simulink model "geometric_control_template_with_estimator"  (R2022b)
settings: Solver=VariableStepAuto  StartTime=0.0  StopTime=120  RelTol=1e-3
InitFcn:
  | %% INITIALIZATION
  | 
  | %% UAV PARAMETERS
  | 
  | mass = 1.2;
  | Ib = diag([1.2416 1.2416 2*1.2416]);
  | g=9.81;
  | e3=[0 0 1]';
  | %% SAMPLING TIME
  | Ts=0.001;
  | 
  | 
  | %data for Simulink
  | pos_0 = [x0 y0 z0];
  | lin_vel_0 = [dot_x0 dot_y0 dot_z0];
  | w_bb_0 = [0 0 0];
  | 
  | %% momentum based estimator param
  | b=50;
  | 
  | r=4; %order of the estimator
  | 
  | 
  | 
  | s=tf('s');
  | G=b^r/(b+s)^r;
  | 
  | c=cell2mat(G.Denominator);
  | 
  | c=c(2:end);
  | 
  | K=zeros(length(r));
  | 
  | P=1; %product of the gains K_i
  | for i=1:r
  |     K(i)=c(i)/P;
  |     P=P*K(i);
  | end
  | K=flip(K);
values from neighbouring files (symbols this model uses):
  dot_x0 = 0    [poly7.m]
  dot_y0 = 0    [poly7.m]
  dot_z0 = 0    [poly7.m]
  i = find(Nodes==Open(1,end))    [DFS.m]
  Track_path = DFS(A_adj,2,path)    [BRRT_3D.m]    (also in GOOD_PATH.mat = [3 15.8545082605 15.9232549014 27.6290043449 38.9996108348 4)
  x0 = pi(1)    [poly7.m]
  y0 = pi(2)    [poly7.m]
  z0 = pi(3)    [poly7.m]
libraries: robotcorelib x1, uavutilslib x1
settings Model: Creator=fabioruggiero  LastModifiedBy=storm
settings ModelReferenceCC: EnableRefExpFcnMdlSchedulingChecks=on

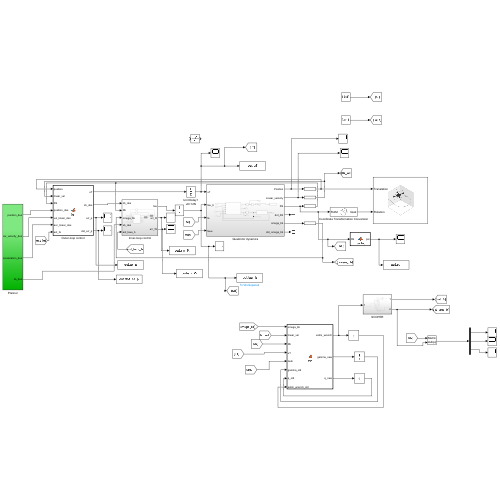
[thumbnail: Simulink's stored preview of the top-level diagram]
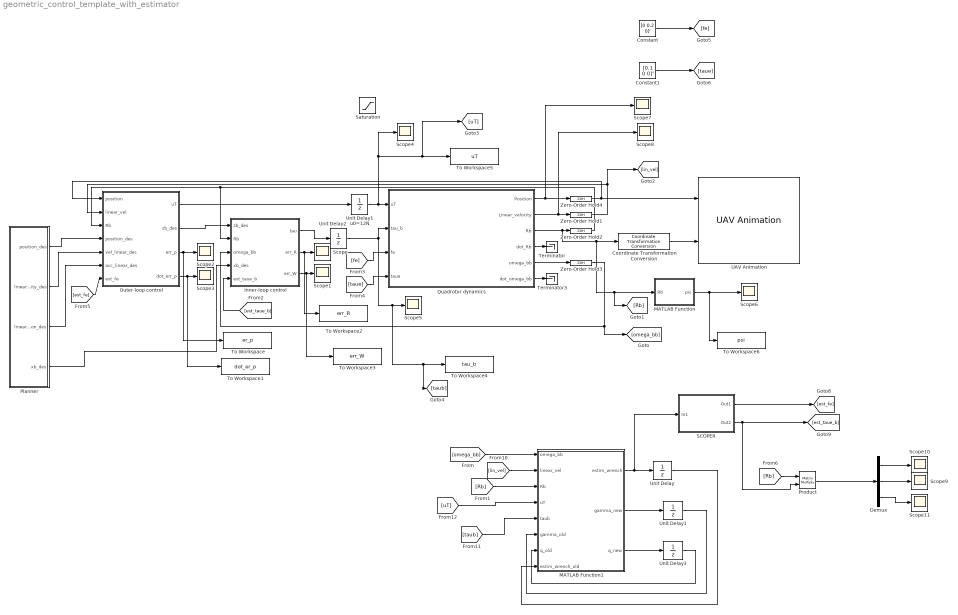
== system geometric_control_template_with_estimator ==
  Constant : Constant  Value=[0 0.2 0]'
  Constant1 : Constant  Value=[0.1 0 0]'
  Coordinate Transformation Conversion : robotcorelib/Coordinate Transformation Conversion  InputRepresentation=Rotation Matrix  InputEulerSequence=ZYX  ShowTrVecInputPort=on  OutputRepresentation=Quaternion  OutputEulerSequence=ZYX  ShowTrVecOutputPort=on  SimulateUsing=Interpreted execution
  Demux : Demux  Outputs=3
  Inner-loop control : Subsystem
  MATLAB Function : MATLAB Function  TreatAsAtomicUnit=on
  MATLAB Function1 : MATLAB Function  TreatAsAtomicUnit=on
  Outer-loop control : MATLAB Function  TreatAsAtomicUnit=on
  Planner : Subsystem
  Product : Product  Multiplication=Matrix(*)
  Quadrotor dynamics : Subsystem
  SCOPER : Subsystem
  Saturation : Saturate  UpperLimit=0.8  LowerLimit=-0.8
  Scope{,1..11} (12 alike) : Scope
  Terminator : Terminator
  Terminator3 : Terminator
  To Workspace : ToWorkspace  VariableName=er_p  SaveFormat=Structure With Time  SampleTime=-1
  To Workspace1 : ToWorkspace  VariableName=dot_er_p  SaveFormat=Structure With Time  SampleTime=-1
  To Workspace2 : ToWorkspace  VariableName=err_R  SaveFormat=Structure With Time  SampleTime=-1
  To Workspace3 : ToWorkspace  VariableName=err_W  SaveFormat=Structure With Time  SampleTime=-1
  To Workspace4 : ToWorkspace  VariableName=tau_b  SaveFormat=Structure With Time  SampleTime=-1
  To Workspace5 : ToWorkspace  VariableName=uT  SaveFormat=Structure With Time  SampleTime=-1
  To Workspace6 : ToWorkspace  VariableName=psi  SaveFormat=Structure With Time  SampleTime=-1
  UAV Animation : uavutilslib/UAV Animation  UAVType=Multirotor  UAVSize=1  InertialZDirection=Down  SampleTime=0.01
  Unit Delay : UnitDelay  InitialCondition=zeros(6,1)  SampleTime=Ts  HasFrameUpgradeWarning=on
  Unit Delay1 : UnitDelay  InitialCondition=zeros(6,r)  SampleTime=Ts  HasFrameUpgradeWarning=on
  Unit Delay1 u0=12N : UnitDelay  InitialCondition=mass*9.81  SampleTime=Ts
  Unit Delay2 : UnitDelay  InitialCondition=[0 0 0]  SampleTime=Ts
  Unit Delay3 : UnitDelay  InitialCondition=zeros(6,1)  SampleTime=Ts  HasFrameUpgradeWarning=on
  Zero-Order Hold{1..4} (4 alike) : ZeroOrderHold  SampleTime=Ts
  wires:
  Outer-loop control/1(uT) -> Unit Delay1 u0=12N/1
  Unit Delay1 u0=12N/1 -> Quadrotor dynamics/1(uT), Scope4/1, [uT], To Workspace5/1
  Quadrotor dynamics/1(Position) -> Scope7/1, Zero-Order Hold4/1
  Quadrotor dynamics/2(Linear_velocity) -> Scope8/1, Zero-Order Hold1/1
  Quadrotor dynamics/3(Rb) -> [Rb], MATLAB Function/1(Rb), Coordinate Transformation Conversion/1, Zero-Order Hold2/1
  Quadrotor dynamics/5(omega_bb) -> Zero-Order Hold3/1
  Zero-Order Hold4/1 -> UAV Animation/1, Outer-loop control/1(position)
  Zero-Order Hold1/1 -> [lin_vel], Outer-loop control/2(linear_vel)
  Zero-Order Hold2/1 -> Outer-loop control/3(Rb), Inner-loop control/2(Rb)
  Quadrotor dynamics/4(dot_Rb) -> Terminator/1
  Planner/1(position_des) -> Outer-loop control/4(position_des)
  Planner/2(linear_velocity_des) -> Outer-loop control/5(vel_linear_des)
  Planner/3(linear_acceleration_des) -> Outer-loop control/6(acc_linear_des)
  Planner/4(xb_des) -> Inner-loop control/4(xb_des)
  Outer-loop control/3(err_p) -> To Workspace/1, Scope2/1
  Outer-loop control/4(dot_err_p) -> To Workspace1/1, Scope3/1
  Quadrotor dynamics/6(dot_omega_bb) -> Terminator3/1
  Coordinate Transformation Conversion/1 -> UAV Animation/2
  Outer-loop control/2(zb_des) -> Inner-loop control/1(zb_des)
  Inner-loop control/1(tau) -> Unit Delay2/1
  Inner-loop control/2(err_R) -> To Workspace2/1, Scope/1
  Inner-loop control/3(err_W) -> To Workspace3/1, Scope1/1
  MATLAB Function/1(psi) -> To Workspace6/1, Scope6/1
  MATLAB Function1/2(gamma_new) -> Unit Delay1/1
  Unit Delay/1 -> MATLAB Function1/8(estim_wrench_old)
  [lin_vel] -> MATLAB Function1/2(linear_vel)
  MATLAB Function1/1(estim_wrench) -> SCOPER/1(In1), Unit Delay/1
  [uT] -> MATLAB Function1/4(uT)
  [taub] -> MATLAB Function1/5(taub)
  Unit Delay1/1 -> MATLAB Function1/6(gamma_old)
  Unit Delay3/1 -> MATLAB Function1/7(q_old)
  SCOPER/2(Out2) -> Product/2, [est_taue_b]
  [omega_bb] -> MATLAB Function1/1(omega_bb)
  SCOPER/1(Out1) -> [est_fe]
  MATLAB Function1/3(q_new) -> Unit Delay3/1
  Zero-Order Hold3/1 -> [omega_bb], Inner-loop control/3(omega_bb)
  [Rb] -> MATLAB Function1/3(Rb)
  [est_taue_b] -> Inner-loop control/5(est_taue_b)
  Constant/1 -> [fe]
  Constant1/1 -> [taue]
  [fe] -> Quadrotor dynamics/3(fe)
  [taue] -> Quadrotor dynamics/4(taue)
  [est_fe] -> Outer-loop control/7(est_fe)
  [Rb] -> Product/1
  Demux/1 -> Scope10/1
  Demux/3 -> Scope11/1
  Demux/2 -> Scope9/1
  Product/1 -> Demux/1
  Unit Delay2/1 -> [taub], To Workspace4/1, Scope5/1, Quadrotor dynamics/2(tau_b)

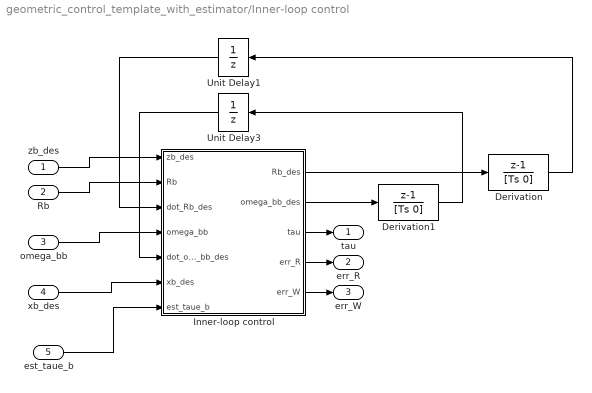
== system geometric_control_template_with_estimator/Inner-loop control ==
  zb_des : Inport
  Rb : Inport  Port=2
  omega_bb : Inport  Port=3
  xb_des : Inport  Port=4
  est_taue_b : Inport  Port=5
  Derivation : DiscreteTransferFcn  Numerator=[1 -1]  Denominator=[Ts 0]  InitialStates=[1 0 0;0 1 0;0 0 1]  SampleTime=Ts
  Derivation1 : DiscreteTransferFcn  Numerator=[1 -1]  Denominator=[Ts 0]  InitialStates=[0 0 0]  SampleTime=Ts
  Inner-loop control : MATLAB Function  TreatAsAtomicUnit=on
  Unit Delay1 : UnitDelay  InitialCondition=eye(3)  SampleTime=Ts
  Unit Delay3 : UnitDelay  InitialCondition=[0 0 0]  SampleTime=Ts
  tau : Outport
  err_R : Outport  Port=2
  err_W : Outport  Port=3
  wires:
  xb_des/1 -> Inner-loop control/6(xb_des)
  Inner-loop control/4(err_R) -> err_R/1
  Rb/1 -> Inner-loop control/2(Rb)
  Inner-loop control/3(tau) -> tau/1
  Unit Delay1/1 -> Inner-loop control/3(dot_Rb_des)
  Derivation1/1 -> Unit Delay3/1
  Inner-loop control/5(err_W) -> err_W/1
  Unit Delay3/1 -> Inner-loop control/5(dot_omega_bb_des)
  Derivation/1 -> Unit Delay1/1
  zb_des/1 -> Inner-loop control/1(zb_des)
  omega_bb/1 -> Inner-loop control/4(omega_bb)
  Inner-loop control/1(Rb_des) -> Derivation/1
  Inner-loop control/2(omega_bb_des) -> Derivation1/1
  est_taue_b/1 -> Inner-loop control/7(est_taue_b)

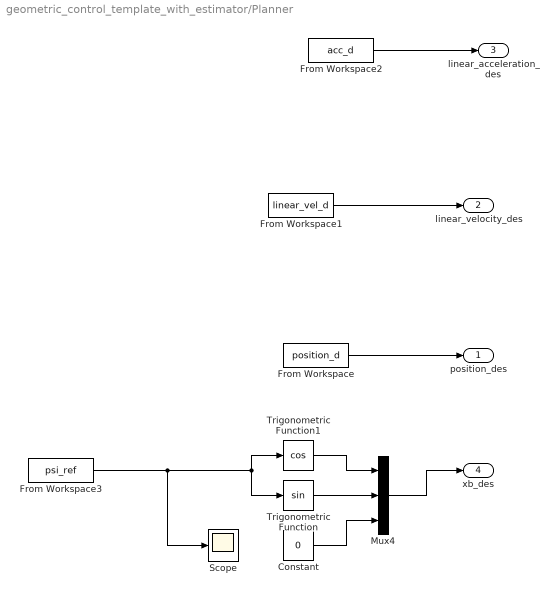
== system geometric_control_template_with_estimator/Planner ==
  Constant : Constant  Value=0
  From Workspace : FromWorkspace  VariableName=position_d
  From Workspace1 : FromWorkspace  VariableName=linear_vel_d
  From Workspace2 : FromWorkspace  VariableName=acc_d
  From Workspace3 : FromWorkspace  VariableName=psi_ref
  Mux4 : Mux  Inputs=3
  Scope : Scope
  Trigonometric Function : Trigonometry
  Trigonometric Function1 : Trigonometry  Operator=cos
  position_des : Outport
  linear_velocity_des : Outport  Port=2
  linear_acceleration_des : Outport  Port=3
  xb_des : Outport  Port=4
  wires:
  Mux4/1 -> xb_des/1
  Trigonometric Function/1 -> Mux4/2
  From Workspace3/1 -> Trigonometric Function/1, Trigonometric Function1/1, Scope/1
  Trigonometric Function1/1 -> Mux4/1
  Constant/1 -> Mux4/3
  From Workspace2/1 -> linear_acceleration_des/1
  From Workspace1/1 -> linear_velocity_des/1
  From Workspace/1 -> position_des/1

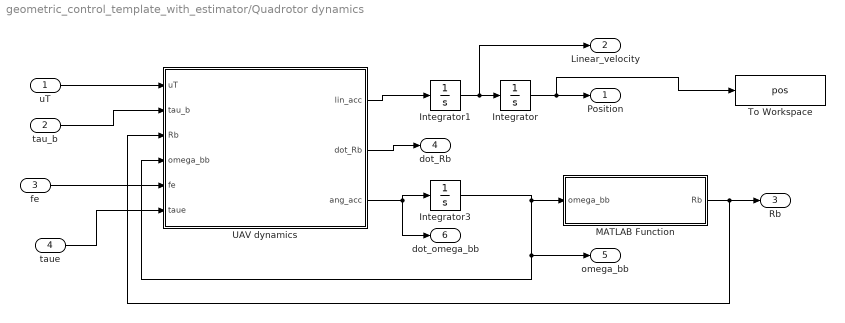
== system geometric_control_template_with_estimator/Quadrotor dynamics ==
  uT : Inport
  tau_b : Inport  Port=2
  fe : Inport  Port=3
  taue : Inport  Port=4
  Integrator : Integrator  InitialCondition=Track_path(1,:)
  Integrator1 : Integrator  InitialCondition=lin_vel_0
  Integrator3 : Integrator  InitialCondition=w_bb_0
  MATLAB Function : MATLAB Function  TreatAsAtomicUnit=on
  To Workspace : ToWorkspace  VariableName=pos  SaveFormat=Structure With Time  SampleTime=-1
  UAV dynamics : MATLAB Function  TreatAsAtomicUnit=on
  Position : Outport
  Linear_velocity : Outport  Port=2
  Rb : Outport  Port=3
  dot_Rb : Outport  Port=4
  omega_bb : Outport  Port=5
  dot_omega_bb : Outport  Port=6
  wires:
  tau_b/1 -> UAV dynamics/2(tau_b)
  UAV dynamics/3(ang_acc) -> Integrator3/1, dot_omega_bb/1
  UAV dynamics/1(lin_acc) -> Integrator1/1
  uT/1 -> UAV dynamics/1(uT)
  Integrator1/1 -> Linear_velocity/1, Integrator/1
  Integrator3/1 -> MATLAB Function/1(omega_bb), UAV dynamics/4(omega_bb), omega_bb/1
  UAV dynamics/2(dot_Rb) -> dot_Rb/1
  MATLAB Function/1(Rb) -> Rb/1, UAV dynamics/3(Rb)
  Integrator/1 -> To Workspace/1, Position/1
  fe/1 -> UAV dynamics/5(fe)
  taue/1 -> UAV dynamics/6(taue)

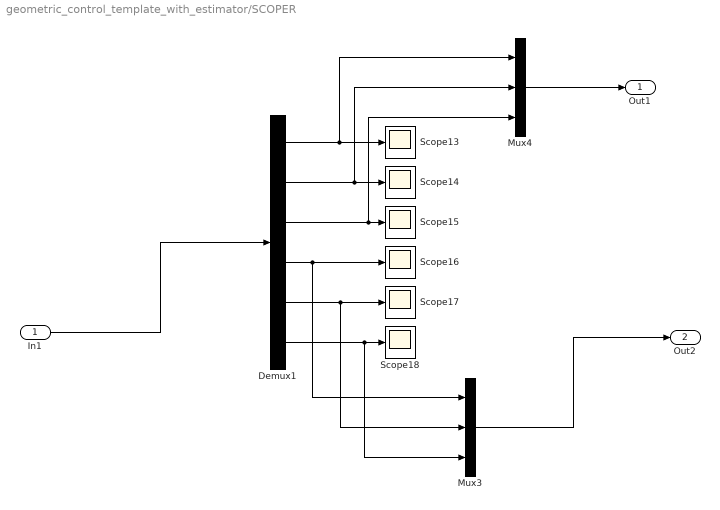
== system geometric_control_template_with_estimator/SCOPER ==
  In1 : Inport
  Demux1 : Demux  Outputs=6
  Mux3 : Mux  Inputs=3
  Mux4 : Mux  Inputs=3
  Scope{13..18} (6 alike) : Scope
  Out1 : Outport
  Out2 : Outport  Port=2
  wires:
  In1/1 -> Demux1/1
  Mux4/1 -> Out1/1
  Demux1/3 -> Mux4/3, Scope15/1
  Demux1/5 -> Mux3/2, Scope17/1
  Demux1/2 -> Mux4/2, Scope14/1
  Demux1/1 -> Mux4/1, Scope13/1
  Demux1/4 -> Mux3/1, Scope16/1
  Demux1/6 -> Mux3/3, Scope18/1
  Mux3/1 -> Out2/1

== matlab function geometric_control_template_with_estimator/Quadrotor dynamics/MATLAB Function ==
  data: omega_bb input; Rb output
function Rb = fcn(omega_bb)

Rb = expm(skew(omega_bb));
end

function S = skew(v)
if(numel(v)~= 1)
S= [0 -v(3) v(2); 
    v(3) 0 -v(1);
    -v(2) v(1) 0];
else
S= zeros(3);
end
end

== matlab function geometric_control_template_with_estimator/Quadrotor dynamics/UAV dynamics ==
  data: uT input size=1; tau_b input size=3; lin_acc output size=3; Rb input size=[3,3]; omega_bb input size=3; dot_Rb output size=[3,3]; ang_acc output size=3; mass parameter size=1; Ib parameter size=[3,3]; fe input; taue input
function [lin_acc, dot_Rb, ang_acc] = fcn(uT,tau_b,Rb,omega_bb,mass, Ib,fe,taue)

lin_acc = 9.81*[0 0 1]'-(uT/mass)*Rb*[0 0 1]'+fe/mass;
dot_Rb = Rb*skew(omega_bb);
ang_acc = inv(Ib)*(-skew(omega_bb)*Ib*omega_bb + tau_b+Rb'*taue);

end

function S = skew(v)
if(numel(v)~= 1)
S= [0 -v(3) v(2); 
    v(3) 0 -v(1);
    -v(2) v(1) 0];
else
S= zeros(3);
end
end

== matlab function geometric_control_template_with_estimator/Outer-loop control ==
  data: position input size=3; uT output size=1; linear_vel input size=3; Rb input size=[3,3]; zb_des output size=3; mass parameter size=1; position_des input size=3; vel_linear_des input size=3; acc_linear_des input size=3; err_p output size=3; dot_err_p output size=3; est_fe input
function [uT, zb_des, err_p, dot_err_p] = fcn(position, linear_vel, Rb, mass, ...
    position_des, vel_linear_des, acc_linear_des,est_fe)

%% WRITE HERE THE OUTER-LOOP CONTROL
% position: linear position measure
% linear_vel: linear velocity measure
% Rb: current rotation matrix
% mass: mass of the UAV
% positon_des: desired linear position from the planner
% vel_linear_des: desired linear velocity from the planner
% acc_linear_des: desired linear acceleration from the planner
% ---
% uT: commanded total thrust
% zb_des: desired z-axis of the body frame
% err_p: position error
% dot_err_p: time derivative of the positon error
Kp=80;
Kv=diag([1 1 5]);
g=9.81;
e3=[0 0 1]';

err_p=position-position_des;
dot_err_p=linear_vel-vel_linear_des;

uT=-(-Kp*err_p-Kv*dot_err_p-mass*g*e3+mass*acc_linear_des-est_fe)'*Rb*e3;

zb_des=-(-Kp*err_p-Kv*dot_err_p-mass*g*e3+mass*acc_linear_des-est_fe)/(norm(-Kp*err_p-Kv*dot_err_p-mass*g*e3+mass*acc_linear_des-est_fe));

end

== matlab function geometric_control_template_with_estimator/Inner-loop control/Inner-loop control ==
  data: Rb_des output size=[3,3]; omega_bb_des output size=3; tau output size=3; zb_des input size=3; Rb input size=[3,3]; dot_Rb_des input size=[3,3]; omega_bb input size=3; dot_omega_bb_des input size=3; xb_des input size=3; Ib parameter size=[3,3]; err_R output size=3; err_W output size=3; est_taue_b input
function [Rb_des,omega_bb_des,tau,err_R,err_W] = fcn(zb_des,Rb,dot_Rb_des,omega_bb,dot_omega_bb_des,xb_des,Ib,est_taue_b)

%% WRITE HERE THE INNER-LOOP CONTROL
% zb_des: desired z-axis of the body frame
% Rb: current rotation matrix
% dot_Rb_des: time-derivative of the desired rotation matrix
% omega_bb: current angular velocity expressed in the body frame
% dot_omega_bb_des: desired angular acceleration expressed in the body
% frame
% xb_des: desired x-axis of the body frame form the planner
% Ib: inertia matrix of the UAV with respect to the body frame
% ---
% Rb_des: desired rotation matrix
% omega_bb_des: desired angular velocity expressed in the body frame (given
% below as a hint)
% tau: commanded control torque
% err_R: rotational error in SO(3)
% err_W: angular velocity error in SO(3)
yb_des=(skew(zb_des)*xb_des)/(norm(skew(zb_des)*xb_des));

Rb_des=[skew(yb_des)*zb_des yb_des zb_des];

omega_bb_des = wedge(Rb_des'*dot_Rb_des);


Kr=50;
Kw=10;


err_R=0.5*wedge(Rb_des'*Rb-Rb'*Rb_des);
err_W=omega_bb-Rb'*Rb_des*omega_bb_des;

tau=-Kr*err_R-Kw*err_W+skew(omega_bb)*Ib*omega_bb-Ib*(skew(omega_bb)*Rb'*Rb_des*omega_bb_des-Rb'*Rb_des*dot_omega_bb_des)-est_taue_b;

end

function S = skew(v)
if(numel(v)~= 1)
S= [0 -v(3) v(2); 
    v(3) 0 -v(1);
    -v(2) v(1) 0];
else
S= zeros(3);
end
end

function v = wedge(S)
v1 = S(3,2);
v2 = S(1,3);
v3 = S(2,1);
v = [v1 v2 v3]';
end

== matlab function geometric_control_template_with_estimator/MATLAB Function ==
  data: Rb input; psi output
function psi = heading(Rb)

psi = rad2deg(atan(Rb(2,1)/Rb(1,1)));

== matlab function geometric_control_template_with_estimator/MATLAB Function1 ==
  data: omega_bb input; linear_vel input; estim_wrench output; Rb input; uT input; taub input; gamma_new output; q_new output; gamma_old input; q_old input; estim_wrench_old input; mass parameter; Ib parameter; r parameter; K parameter; Ts parameter; g parameter; e3 parameter
function [estim_wrench, gamma_new, q_new] = fcn(omega_bb,linear_vel,Rb,uT,taub,gamma_old,q_old,estim_wrench_old, mass, Ib,r, K,Ts,g, e3)
    
    
    
    q_new=[mass*eye(3) zeros(3,3);zeros(3,3) Ib]*[linear_vel;omega_bb];

    gamma_new=gamma_old;
    gamma_new(:,1)=gamma_old(:,1)+K(1)*((q_new-q_old)-Ts*[mass*g*e3-uT*Rb*e3;-skew(omega_bb)*Ib*omega_bb+taub]-Ts*estim_wrench_old);
    
    if r>=2
        for i=2:r
            
            gamma_new(:,i)=gamma_old(:,i)+Ts*K(i)*(-estim_wrench_old+gamma_old(:,i-1));

        end
        
    end
    estim_wrench=gamma_new(:,r);



end




function S=skew(w)

if(numel(w)~= 1)

S= [0 -w(3) w(2);
w(3) 0 -w(1);
-w(2) w(1) 0];

else

S= zeros(3);

end

end
